simulink model "hmi_ut"  (Simulink 8.1)
settings: Solver=FixedStepDiscrete  StartTime=0.0  StopTime=10.0  FixedStep=0.005  RelTol=1e-3
libraries: siltestlib x39, hmi x1
settings Model: Creator=AT015555  LastModifiedBy=AT015555
settings DataIOCC: SignalLoggingSaveFormat=Dataset
settings OptimizationCC: ExpressionDepthLimit=128
settings DebuggingCC: FcnCallInpInsideContextMsg=EnableAllAsError
settings GRTTargetCC: CombineOutputUpdateFcns=on  GRTInterface=off

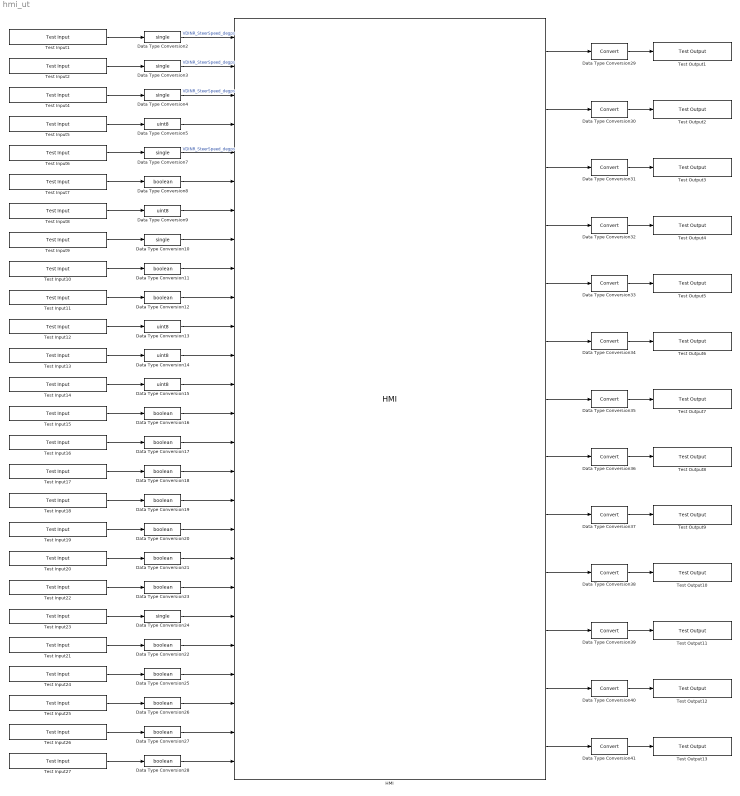
== system hmi_ut ==
  Data Type Conversion{2..4,7,10,24} (6 alike) : DataTypeConversion  OutDataTypeStr=single
  Data Type Conversion{8,11..12,16..23,25..28} (15 alike) : DataTypeConversion  OutDataTypeStr=boolean
  Data Type Conversion{5,9,13..15} (5 alike) : DataTypeConversion  OutDataTypeStr=uint8
  Data Type Conversion{29..41} (13 alike) : DataTypeConversion
  HMI : hmi/HMI
  Test Input1 : siltestlib/Test Input  varname=VDINR_SteerAngle_deg  sampletime=0.005
  Test Input10 : siltestlib/Test Input  varname=VDINR_ACCOnVCU_flg  sampletime=0.005
  Test Input11 : siltestlib/Test Input  varname=VDINR_TurnSignalSwL_flg  sampletime=0.005
  Test Input12 : siltestlib/Test Input  varname=VFCW_FCWStateHMIPrev_enum  sampletime=0.005
  Test Input13 : siltestlib/Test Input  varname=VAEB_AEBStateHMIPrev_enum  sampletime=0.005
  Test Input14 : siltestlib/Test Input  varname=VACC_ACCSytemStatePrev_enum  sampletime=0.005
  Test Input15 : siltestlib/Test Input  varname=VACC_ACCActingPrev_flg  sampletime=0.005
  Test Input16 : siltestlib/Test Input  varname=VDINR_ACCSetSpdDecH_flg  sampletime=0.005
  Test Input17 : siltestlib/Test Input  varname=VDINR_ACCSpdDecH_flg  sampletime=0.005
  Test Input18 : siltestlib/Test Input  varname=VDINR_ACCSetSpdDecVCU_flg  sampletime=0.005
  Test Input19 : siltestlib/Test Input  varname=VDINR_ACCResSpdIncH_flg  sampletime=0.005
  Test Input2 : siltestlib/Test Input  varname=VDINR_SteerSpeed_degps  sampletime=0.005
  Test Input20 : siltestlib/Test Input  varname=VDINR_ACCSpdIncH_flg  sampletime=0.005
  Test Input21 : siltestlib/Test Input  varname=VDINR_ACCResSpdIncVCU_flg  sampletime=0.005
  Test Input22 : siltestlib/Test Input  varname=VIFO_ACCTargetVehAssigned_flg  sampletime=0.005
  Test Input23 : siltestlib/Test Input  varname=VJUD_ACCSetSpeedPrev_kph  sampletime=0.005
  Test Input24 : siltestlib/Test Input  varname=VDINR_ACCDistVCU_flg  sampletime=0.005
  Test Input25 : siltestlib/Test Input  varname=VDINR_ACCTimeGapDecH_flg  sampletime=0.005
  Test Input26 : siltestlib/Test Input  varname=VDINR_ACCOnH_flg  sampletime=0.005
  Test Input27 : siltestlib/Test Input  varname=VDINR_TurnSignalSwR_flg  sampletime=0.005
  Test Input4 : siltestlib/Test Input  varname=VDINR_HWAccelPedalPosn_pct  sampletime=0.005
  Test Input5 : siltestlib/Test Input  varname=VDINR_ParkBrakeBindSta_enum  sampletime=0.005
  Test Input6 : siltestlib/Test Input  varname=VDINR_MCPressure_bar  sampletime=0.005
  Test Input7 : siltestlib/Test Input  varname=VDINR_DriverBrakPedalOn_flg  sampletime=0.005
  Test Input8 : siltestlib/Test Input  varname=VDINR_NowGearPosn_enum  sampletime=0.005
  Test Input9 : siltestlib/Test Input  varname=VDINR_VehSpd_mps  sampletime=0.005
  Test Output1 : siltestlib/Test Output  varname=VIFO_DriverOverrideReq_flg  sampletime=-1
  Test Output10 : siltestlib/Test Output  varname=VIFO_ACCSetSpdDec_flg  sampletime=-1
  Test Output11 : siltestlib/Test Output  varname=VIFO_ACCResSpdInc_flg  sampletime=-1
  Test Output12 : siltestlib/Test Output  varname=VIFO_ACCDist_flg  sampletime=-1
  Test Output13 : siltestlib/Test Output  varname=VIFO_DriverTurnSignalOn_flg  sampletime=-1
  Test Output2 : siltestlib/Test Output  varname=VIFO_AggressiveDriverDetec_flg  sampletime=-1
  Test Output3 : siltestlib/Test Output  varname=VIFO_ActiveDriverDetec_flg  sampletime=-1
  Test Output4 : siltestlib/Test Output  varname=VIFO_ParkingSituation_flg  sampletime=-1
  Test Output5 : siltestlib/Test Output  varname=VIFO_BrakePedalPressed_flg  sampletime=-1
  Test Output6 : siltestlib/Test Output  varname=VIFO_ACCTurnOnReq_flg  sampletime=-1
  Test Output7 : siltestlib/Test Output  varname=VIFO_ACCTurnOffReq_flg  sampletime=-1
  Test Output8 : siltestlib/Test Output  varname=VIFO_ACCCancelReq_flg  sampletime=-1
  Test Output9 : siltestlib/Test Output  varname=VIFO_DriverOvertakeReq_flg  sampletime=-1
  wires:
  Test Input1/1 -> Data Type Conversion2/1
  Data Type Conversion2/1 -> HMI/1  "VDINR_SteerSpeed_degps"
  Test Input2/1 -> Data Type Conversion3/1
  Data Type Conversion3/1 -> HMI/2  "VDINR_SteerSpeed_degps"
  Test Input4/1 -> Data Type Conversion4/1
  Data Type Conversion4/1 -> HMI/3  "VDINR_SteerSpeed_degps"
  Test Input5/1 -> Data Type Conversion5/1
  Data Type Conversion5/1 -> HMI/4
  Test Input6/1 -> Data Type Conversion7/1
  Data Type Conversion7/1 -> HMI/5  "VDINR_SteerSpeed_degps"
  Test Input7/1 -> Data Type Conversion8/1
  Test Input8/1 -> Data Type Conversion9/1
  Test Input9/1 -> Data Type Conversion10/1
  Test Input10/1 -> Data Type Conversion11/1
  Test Input11/1 -> Data Type Conversion12/1
  Test Input12/1 -> Data Type Conversion13/1
  Test Input13/1 -> Data Type Conversion14/1
  Test Input14/1 -> Data Type Conversion15/1
  Test Input15/1 -> Data Type Conversion16/1
  Test Input16/1 -> Data Type Conversion17/1
  Test Input17/1 -> Data Type Conversion18/1
  Test Input18/1 -> Data Type Conversion19/1
  Test Input19/1 -> Data Type Conversion20/1
  Test Input20/1 -> Data Type Conversion21/1
  Test Input21/1 -> Data Type Conversion22/1
  Test Input22/1 -> Data Type Conversion23/1
  Test Input23/1 -> Data Type Conversion24/1
  Test Input24/1 -> Data Type Conversion25/1
  Test Input25/1 -> Data Type Conversion26/1
  Test Input26/1 -> Data Type Conversion27/1
  Test Input27/1 -> Data Type Conversion28/1
  Data Type Conversion8/1 -> HMI/6
  Data Type Conversion21/1 -> HMI/19
  Data Type Conversion22/1 -> HMI/22
  Data Type Conversion9/1 -> HMI/7
  Data Type Conversion20/1 -> HMI/18
  Data Type Conversion17/1 -> HMI/15
  Data Type Conversion12/1 -> HMI/10
  Data Type Conversion18/1 -> HMI/16
  Data Type Conversion16/1 -> HMI/14
  Data Type Conversion11/1 -> HMI/9
  Data Type Conversion15/1 -> HMI/13
  Data Type Conversion19/1 -> HMI/17
  Data Type Conversion14/1 -> HMI/12
  Data Type Conversion10/1 -> HMI/8
  Data Type Conversion13/1 -> HMI/11
  Data Type Conversion27/1 -> HMI/25
  Data Type Conversion28/1 -> HMI/26
  Data Type Conversion26/1 -> HMI/24
  Data Type Conversion24/1 -> HMI/21
  Data Type Conversion25/1 -> HMI/23
  Data Type Conversion23/1 -> HMI/20
  Data Type Conversion29/1 -> Test Output1/1
  HMI/1 -> Data Type Conversion29/1
  Data Type Conversion30/1 -> Test Output2/1
  Data Type Conversion31/1 -> Test Output3/1
  HMI/2 -> Data Type Conversion30/1
  HMI/3 -> Data Type Conversion31/1
  Data Type Conversion32/1 -> Test Output4/1
  HMI/4 -> Data Type Conversion32/1
  Data Type Conversion33/1 -> Test Output5/1
  HMI/5 -> Data Type Conversion33/1
  Data Type Conversion34/1 -> Test Output6/1
  HMI/6 -> Data Type Conversion34/1
  Data Type Conversion35/1 -> Test Output7/1
  HMI/7 -> Data Type Conversion35/1
  Data Type Conversion36/1 -> Test Output8/1
  HMI/8 -> Data Type Conversion36/1
  Data Type Conversion37/1 -> Test Output9/1
  Data Type Conversion38/1 -> Test Output10/1
  HMI/9 -> Data Type Conversion37/1
  HMI/10 -> Data Type Conversion38/1
  Data Type Conversion39/1 -> Test Output11/1
  HMI/11 -> Data Type Conversion39/1
  Data Type Conversion40/1 -> Test Output12/1
  HMI/12 -> Data Type Conversion40/1
  Data Type Conversion41/1 -> Test Output13/1
  HMI/13 -> Data Type Conversion41/1
